simulink model "hw3_eye_prob4"  (R2017a)
settings: Solver=ode45  StartTime=0.0  StopTime=0.5  FixedStep=.0001  MaxStep=.002  RelTol=1e-3  EnableMultiTasking=on
undefined symbols (not defined in the file or in its folder): sigbuilder_block
settings Model: Creator=wintersj  LastModifiedBy=JP
settings DataIOCC: LimitDataPoints=on  SaveFormat=Array  SignalLoggingSaveFormat=ModelDataLogs
settings OptimizationCC: ExpressionDepthLimit=2147483647  LifeSpan=inf
settings DebuggingCC: UnderspecifiedInitializationDetection=Classic  MergeDetectMultiDrivingBlocksExec=none  MaxConsecutiveZCsMsg=none  SolverPrmCheckMsg=warning  FcnCallInpInsideContextMsg=warning  StateNameClashWarn=warning  SFUnexpectedBacktrackingDiag=warning  SFNoUnconditionalDefaultTransitionDiag=warning  SFExecutionAtInitializationDiag=none
settings HardwareCC: ProdBitPerPointer=32  ProdBitPerSizeT=32  ProdBitPerPtrDiffT=32  ProdLargestAtomicFloat=None  ProdIntDivRoundTo=Undefined  ProdEndianess=Unspecified  ProdWordSize=32  ProdHWDeviceType=32-bit Generic
settings ModelReferenceCC: PropagateSignalLabelsOutOfModel=off
settings GRTTargetCC: TargetLangStandard=C89/C90 (ANSI)  GeneratePreprocessorConditionals=Disable all  CombineOutputUpdateFcns=off  GRTInterface=on
settings ConfigComp: CovMetricSettings=dw  CovHtmlReporting=on  CovSaveCumulativeToWorkspaceVar=on  CovSaveSingleToWorkspaceVar=on  CovExternalEMLEnable=off

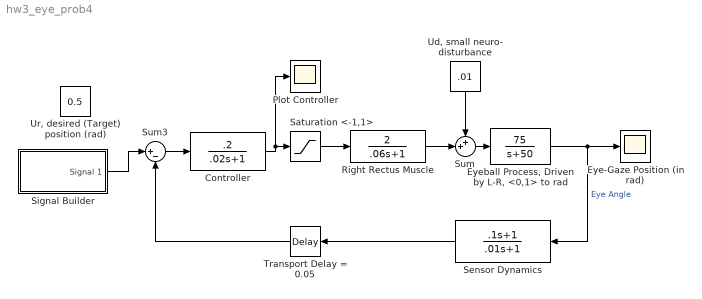
== system hw3_eye_prob4 ==
  Controller : TransferFcn  Numerator=[.2]  Denominator=[.02 1]
  Eye-Gaze Position (in rad) : Scope
  "Eyeball Process, Driven by L-R, <0,1> to rad" : TransferFcn  Numerator=[75]  Denominator=[1 50]
  "Plot Controller " : Scope
  Right Rectus Muscle : TransferFcn  Numerator=[2]  Denominator=[.06 1]
  Saturation <-1,1> : Saturate  UpperLimit=1  LowerLimit=-1
  Sensor Dynamics : TransferFcn  Numerator=[.1 1]  Denominator=[.01 1]
  Signal Builder : Subsystem  Tag=STV Subsys  LoadFcn=sigbuilder_block('load',[437.6 199.2 550.4 400 ]);  StartFcn=sigbuilder_block('start');  StopFcn=sigbuilder_block('stop');  ClipboardFcn=sigbuilder_block('clipboard');  mask(Sigbuilder block){tuvar=[0:10]}
      mask help: Simulink:masks:SigbuilderBlock_MD
      mask init:
      | if ~strcmp(get_param(bdroot(gcbh),'SimulationStatus'),'stopped') tuvar = sigbuilder_block('maskInit'); end
      settings: CopyFcn=sigbuilder_block('copy');  DeleteFcn=sigbuilder_block('delete');  ModelCloseFcn=sigbuilder_block('modelClose');  PreSaveFcn=sigbuilder_block('preSave');  PauseFcn=sigbuilder_block('pause');  ContinueFcn=sigbuilder_block('continue');  NameChangeFcn=sigbuilder_block('namechange');  OpenFcn=sigbuilder_block('open',[437.6 199.2 550.4 400 ]);  CloseFcn=sigbuilder_block('close');
      mask Display: plot(0, 0, 100, 100,[2, 2, 32, 32, 2], [68, 8, 8, 68, 68],[32, 2], [38, 38], [32, 19, 2],[53, 60, 44], [32, 17, 17, 2],[16, 16, 31, 31]);txt = getActiveGroup(gcbh);text(2, 100, txt,'verticalAlignment', 'top');
  Sum : Sum  Inputs=++|
  Sum3 : Sum  Inputs=|+-
  Transport Delay = 0.05 : TransportDelay  DelayTime=.05
  "Ud, small neuro- disturbance" : Constant  Value=.01
  "Ur, desired (Target) position (rad)" : Constant  Value=0.5
  wires:
  Sum/1 -> "Eyeball Process, Driven by L-R, <0,1> to rad"/1
  "Eyeball Process, Driven by L-R, <0,1> to rad"/1 -> Eye-Gaze Position (in rad)/1, Sensor Dynamics/1  "Eye Angle"
  "Ud, small neuro- disturbance"/1 -> Sum/1
  Sensor Dynamics/1 -> Transport Delay = 0.05/1
  Transport Delay = 0.05/1 -> Sum3/2
  Right Rectus Muscle/1 -> Sum/2
  Sum3/1 -> Controller/1
  Controller/1 -> "Plot Controller "/1, Saturation <-1,1>/1
  Saturation <-1,1>/1 -> Right Rectus Muscle/1
  Signal Builder/1(Signal 1) -> Sum3/1

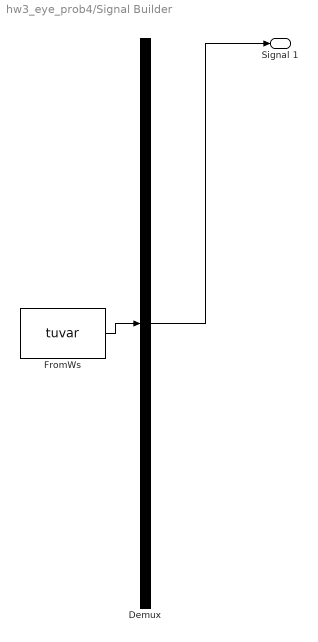
== system hw3_eye_prob4/Signal Builder ==
  Demux : Demux  Tag=STV Demux  Outputs=1
  FromWs : FromWorkspace  Tag=STV FromWs  VariableName=tuvar  SampleTime=0
      SigBuilderData=|
      | common.afterFinalStr = 'Extrapolate'
      | common.sampleTime = 0
      | dataSet.timeRange = [0 10]
      | dataSet.name = 'Group 1'
      | sbobj.Groups.Name = 'Group 1'
      | sbobj.Groups.Signals.Name = 'Signal 1'
      | sbobj.Groups.Signals.XData = [0 0.05 0.05 0.99 0.99 10]
      | sbobj.Groups.Signals.YData = [1 1 0.5 0.5 0 0]
  Signal 1 : Outport  Tag=STV Outport
  wires:
  Demux/1 -> Signal 1/1
  FromWs/1 -> Demux/1
